simulink model "CACC_4_Robots"  (R2021a)
settings: Solver=FixedStepAuto  StartTime=0.0  StopTime=Tsim  RelTol=1e-3
values from neighbouring files (symbols this model uses):
  h = 1.0    (= 1)    [ros_cacc.m]    (also in ros_cacc2.m)
  k1 = 1    [ros_cacc.m]    (also in ros_cacc2.m)
  k2 = 1    [ros_cacc.m]    (also in ros_cacc2.m)
  r = 1    [ros_cacc.m]    (also in ros_cacc2.m)
  v_0 = 0.5    [ros_cacc.m]    (also in ros_cacc2.m)
  v_threshold = v_thr    (= 0.1)    [ros_cacc.m]    (also in ros_cacc2.m)
undefined symbols (not defined in the file or in its folder): angular, linear
libraries: ros2lib x17, robotcorelib x4
(part 2 of 3)

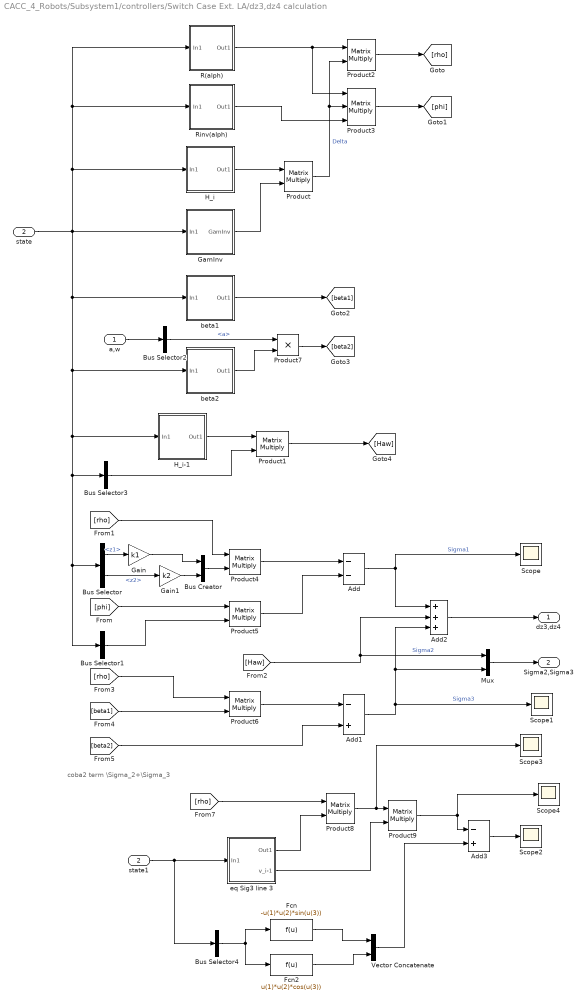
== system CACC_4_Robots/Subsystem1/controllers/Switch Case Ext. LA/dz3,dz4 calculation ==
  note: coba2 term \Sigma_2+\Sigma_3
  a,w : Inport
  state : Inport  Port=2
  Add : Sum  Inputs=--
  Add1 : Sum  Inputs=-+
  Add2 : Sum  Inputs=+++
  Add3 : Sum  Inputs=-+
  Bus Creator : BusCreator  Inputs=2
  Bus Selector : BusSelector  OutputSignals=z1,z2
  Bus Selector1 : BusSelector  OutputSignals=z3,z4  OutputAsBus=on
  Bus Selector2 : BusSelector  OutputSignals=a
  Bus Selector3 : BusSelector  OutputSignals=vdot_ref,thetadot_ref  OutputAsBus=on
  Bus Selector4 : BusSelector  OutputSignals=v_ref,thetadot_ref,theta_ref  OutputAsBus=on
  Fcn : Fcn  Expr=-u(1)*u(2)*sin(u(3))
  Fcn2 : Fcn  Expr=u(1)*u(2)*cos(u(3))
  Gain : Gain  Gain=k1
  Gain1 : Gain  Gain=k2
  "GamInv " : Subsystem
  H_i : Subsystem
  H_i-1 : Subsystem
  Mux : Mux  Inputs=2
  Product{,1..2,4..6,8..9} (8 alike) : Product  Multiplication=Matrix(*)
  Product3 : Product  Inputs=3  Multiplication=Matrix(*)
  Product7 : Product
  R(alph) : Subsystem
  Rinv(alph) : Subsystem
  Scope{,1..4} (5 alike) : Scope
  Vector Concatenate : Concatenate
  beta1 : Subsystem
  beta2 : Subsystem
  eq Sig3 line 3 : Subsystem
  state1 : InportShadow  Port=2
  dz3,dz4 : Outport  VectorParamsAs1DForOutWhenUnconnected=off
  Sigma2,Sigma3 : Outport  Port=2  VectorParamsAs1DForOutWhenUnconnected=off
  wires:
  state/1 -> beta1/1(In1), beta2/1(In1), H_i-1/1(In1), Bus Selector3/1, Bus Selector1/1, Bus Selector/1, Rinv(alph)/1(In1), R(alph)/1(In1), H_i/1(In1), "GamInv "/1(In1)
  H_i-1/1(Out1) -> Product1/1
  H_i/1(Out1) -> Product/1
  "GamInv "/1(GamInv) -> Product/2
  R(alph)/1(Out1) -> Product3/1, Product2/1
  Product/1 -> Product3/2, Product2/2  "Delta"
  Rinv(alph)/1(Out1) -> Product3/3
  Product2/1 -> [rho]
  Product3/1 -> [phi]
  beta1/1(Out1) -> [beta1]
  Product1/1 -> [Haw]
  Bus Selector/1 -> Gain/1  "<z1>"
  Bus Selector/2 -> Gain1/1  "<z2>"
  Gain/1 -> Bus Creator/1
  Gain1/1 -> Bus Creator/2
  Bus Creator/1 -> Product4/2
  [rho] -> Product4/1
  [phi] -> Product5/1
  Bus Selector1/1 -> Product5/2
  Product4/1 -> Add/1
  Product5/1 -> Add/2
  [rho] -> Product6/1
  [beta1] -> Product6/2
  Product6/1 -> Add1/1
  Add/1 -> Add2/1, Scope/1  "Sigma1"
  Add1/1 -> Mux/2, Add2/3, Scope1/1  "Sigma3"
  Add2/1 -> dz3,dz4/1
  a,w/1 -> Bus Selector2/1
  Bus Selector2/1 -> Product7/1  "<a>"
  [Haw] -> Mux/1, Add2/2  "Sigma2"
  Product7/1 -> [beta2]
  beta2/1(Out1) -> Product7/2
  [beta2] -> Add1/2
  Bus Selector3/1 -> Product1/2
  [rho] -> Product8/1
  eq Sig3 line 3/1(Out1) -> Product8/2
  Product8/1 -> Scope3/1, Product9/1
  Vector Concatenate/1 -> Add3/2
  Add3/1 -> Scope2/1
  state1/1 -> Bus Selector4/1, eq Sig3 line 3/1(In1)
  Bus Selector4/1 -> Fcn2/1, Fcn/1
  Fcn/1 -> Vector Concatenate/1
  Fcn2/1 -> Vector Concatenate/2
  eq Sig3 line 3/2(v_i-1) -> Product9/2
  Product9/1 -> Scope4/1, Add3/1
  Mux/1 -> Sigma2,Sigma3/1

== system CACC_4_Robots/Subsystem1/controllers/Switch Case Ext. LA/in parentheses ==
  In1 : Inport
  Add : Sum  Inputs=++++
  Bus Selector : BusSelector  OutputSignals=z1,z2
  Bus Selector1 : BusSelector  OutputSignals=alpha,z3,z4  OutputAsBus=on
  Bus Selector2 : BusSelector  OutputSignals=alpha,v_ref,theta_ref  OutputAsBus=on
  Bus Selector3 : BusSelector  OutputSignals=theta_ref,thetadot_ref,s  OutputAsBus=on
  Fcn : Fcn  Expr=cos(u(1))*u(2)+sin(u(1))*u(3)
  Fcn1 : Fcn  Expr=sin(u(1))*u(2)+cos(u(1))*u(3)
  Fcn2 : Fcn  Expr=(1-cos(u(1)))*u(2)*cos(u(3))-sin(u(1))*u(2)*sin(u(3))
  Fcn3 : Fcn  Expr=sin(u(1))*u(2)*cos(u(3))+(1-cos(u(1)))*u(2)*sin(u(3))
  Fcn4 : Fcn  Expr=cos(u(1))*u(3)*u(2)
  Fcn5 : Fcn  Expr=sin(u(1))*u(3)*u(2)
  Gain : Gain  Gain=k1
  Gain1 : Gain  Gain=k2
  Mux{1..4} (4 alike) : Mux  Inputs=2
  () : Outport  VectorParamsAs1DForOutWhenUnconnected=off
  wires:
  In1/1 -> Bus Selector3/1, Bus Selector2/1, Bus Selector1/1, Bus Selector/1
  Bus Selector/1 -> Gain/1  "<z1>"
  Bus Selector/2 -> Gain1/1  "<z2>"
  Gain/1 -> Mux1/1
  Gain1/1 -> Mux1/2
  Bus Selector1/1 -> Fcn1/1, Fcn/1
  Fcn/1 -> Mux2/1
  Fcn1/1 -> Mux2/2
  Bus Selector2/1 -> Fcn3/1, Fcn2/1
  Fcn2/1 -> Mux3/1
  Fcn3/1 -> Mux3/2
  Bus Selector3/1 -> Fcn5/1, Fcn4/1
  Fcn4/1 -> Mux4/1
  Fcn5/1 -> Mux4/2
  Mux1/1 -> Add/1
  Mux2/1 -> Add/2
  Mux3/1 -> Add/3
  Mux4/1 -> Add/4
  Add/1 -> ()/1

== system CACC_4_Robots/Subsystem1/controllers/Switch Case Ext. LA/invGam ==
  In1 : Inport
  11 : Fcn  Expr=(r+h*u(1))*cos(u(2))
  12 : Fcn  Expr=(r+h*u(1))*sin(u(2))
  21 : Fcn  Expr=-h*sin(u(2))-h*sin(u(13))*cos(u(8))
  22 : Fcn  Expr=h*cos(u(2))-h*sin(u(13))*sin(u(8))
  Divide{,1..3} (4 alike) : Product  Inputs=*/
  Mux : Mux
  det(Gam) : Fcn  Expr=((r+h*u(1))*(h-h*sin(u(13))*sin(u(8)-u(2))))
  invGam : Outport  VectorParamsAs1DForOutWhenUnconnected=off
  wires:
  In1/1 -> 11/1, 12/1, 22/1, det(Gam)/1, 21/1
  Mux/1 -> invGam/1
  11/1 -> Divide/1
  12/1 -> Divide1/1
  21/1 -> Divide2/1
  22/1 -> Divide3/1
  det(Gam)/1 -> Divide2/2, Divide1/2, Divide/2, Divide3/2
  Divide/1 -> Mux/1
  Divide1/1 -> Mux/2
  Divide2/1 -> Mux/3
  Divide3/1 -> Mux/4

== system CACC_4_Robots/Subsystem1/controllers/Switch Case Ext. LA/s ==
  state_prec : Inport
  state : Inport  Port=2
  Approximation of s around zero : Subsystem  TreatAsAtomicUnit=on
  Bus Selector : BusSelector  OutputSignals=curv
  Bus Selector1 : BusSelector  OutputSignals=v
  If : If  IfExpression=u1 < 0.01 & u1 > -0.01
  Merge : Merge
  Mux : Mux  Inputs=2
  function s : Subsystem  TreatAsAtomicUnit=on
  s : Outport  VectorParamsAs1DForOutWhenUnconnected=off
  wires:
  state_prec/1 -> Bus Selector/1
  Bus Selector/1 -> Mux/1, If/1  "<curv>"
  If/1 -> Approximation of s around zero/Action
  If/2 -> function s/Action
  Approximation of s around zero/1(Out1) -> Merge/1
  function s/1(Out1) -> Merge/2
  state/1 -> Bus Selector1/1
  Bus Selector1/1 -> Mux/2  "<v>"
  Mux/1 -> function s/1(In1), Approximation of s around zero/1(In1)
  Merge/1 -> s/1

== system CACC_4_Robots/Subsystem2/controllers/Switch Case Ext. LA/alpha ==
  state_prec : Inport
  state : Inport  Port=2
  Bus Selector : BusSelector  OutputSignals=curv
  Bus Selector1 : BusSelector  OutputSignals=v
  Fcn : Fcn  Expr=atan(u(1)*(r+h*u(2)))
  Mux : Mux  Inputs=2
  alpha : Outport  VectorParamsAs1DForOutWhenUnconnected=off
  wires:
  state_prec/1 -> Bus Selector/1
  state/1 -> Bus Selector1/1
  Mux/1 -> Fcn/1
  Bus Selector/1 -> Mux/1  "<curv>"
  Bus Selector1/1 -> Mux/2  "<v>"
  Fcn/1 -> alpha/1

== system CACC_4_Robots/Subsystem2/controllers/Switch Case Ext. LA/disturbance term simplified ==
  In1 : Inport
  (a,w)ref : Inport  Port=2
  Add : Sum  Inputs=-+
  "GamInv " : Subsystem
  H : Subsystem
  H1 : Subsystem
  Product : Product  Inputs=4  Multiplication=Matrix(*)
  Product1 : Product  Multiplication=Matrix(*)
  R(alph) : Subsystem
  beta1 : Subsystem
  dist1,dist2 : Outport  VectorParamsAs1DForOutWhenUnconnected=off
  wires:
  Add/1 -> dist1,dist2/1
  Product/1 -> Add/1
  (a,w)ref/1 -> Product1/2
  H1/1(Out1) -> Product1/1
  beta1/1(Out1) -> Product/4
  "GamInv "/1(GamInv) -> Product/3
  H/1(Out1) -> Product/2
  R(alph)/1(Out1) -> Product/1
  In1/1 -> H/1(In1), R(alph)/1(In1), "GamInv "/1(In1), beta1/1(In1), H1/1(In1)
  Product1/1 -> Add/2

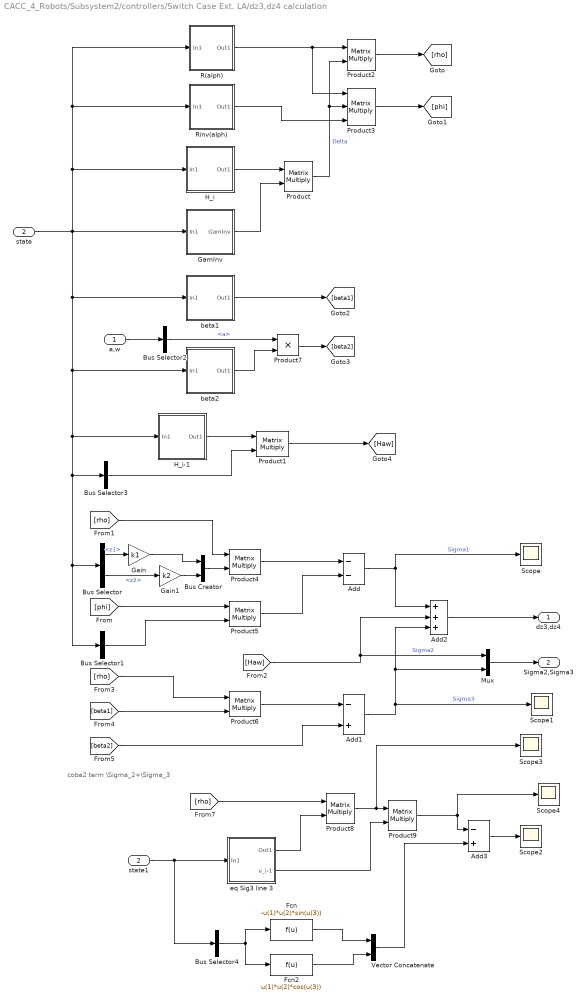
== system CACC_4_Robots/Subsystem2/controllers/Switch Case Ext. LA/dz3,dz4 calculation ==
  note: coba2 term \Sigma_2+\Sigma_3
  a,w : Inport
  state : Inport  Port=2
  Add : Sum  Inputs=--
  Add1 : Sum  Inputs=-+
  Add2 : Sum  Inputs=+++
  Add3 : Sum  Inputs=-+
  Bus Creator : BusCreator  Inputs=2
  Bus Selector : BusSelector  OutputSignals=z1,z2
  Bus Selector1 : BusSelector  OutputSignals=z3,z4  OutputAsBus=on
  Bus Selector2 : BusSelector  OutputSignals=a
  Bus Selector3 : BusSelector  OutputSignals=vdot_ref,thetadot_ref  OutputAsBus=on
  Bus Selector4 : BusSelector  OutputSignals=v_ref,thetadot_ref,theta_ref  OutputAsBus=on
  Fcn : Fcn  Expr=-u(1)*u(2)*sin(u(3))
  Fcn2 : Fcn  Expr=u(1)*u(2)*cos(u(3))
  Gain : Gain  Gain=k1
  Gain1 : Gain  Gain=k2
  "GamInv " : Subsystem
  H_i : Subsystem
  H_i-1 : Subsystem
  Mux : Mux  Inputs=2
  Product{,1..2,4..6,8..9} (8 alike) : Product  Multiplication=Matrix(*)
  Product3 : Product  Inputs=3  Multiplication=Matrix(*)
  Product7 : Product
  R(alph) : Subsystem
  Rinv(alph) : Subsystem
  Scope{,1..4} (5 alike) : Scope
  Vector Concatenate : Concatenate
  beta1 : Subsystem
  beta2 : Subsystem
  eq Sig3 line 3 : Subsystem
  state1 : InportShadow  Port=2
  dz3,dz4 : Outport  VectorParamsAs1DForOutWhenUnconnected=off
  Sigma2,Sigma3 : Outport  Port=2  VectorParamsAs1DForOutWhenUnconnected=off
  wires:
  state/1 -> beta1/1(In1), beta2/1(In1), H_i-1/1(In1), Bus Selector3/1, Bus Selector1/1, Bus Selector/1, Rinv(alph)/1(In1), R(alph)/1(In1), H_i/1(In1), "GamInv "/1(In1)
  H_i-1/1(Out1) -> Product1/1
  H_i/1(Out1) -> Product/1
  "GamInv "/1(GamInv) -> Product/2
  R(alph)/1(Out1) -> Product3/1, Product2/1
  Product/1 -> Product3/2, Product2/2  "Delta"
  Rinv(alph)/1(Out1) -> Product3/3
  Product2/1 -> [rho]
  Product3/1 -> [phi]
  beta1/1(Out1) -> [beta1]
  Product1/1 -> [Haw]
  Bus Selector/1 -> Gain/1  "<z1>"
  Bus Selector/2 -> Gain1/1  "<z2>"
  Gain/1 -> Bus Creator/1
  Gain1/1 -> Bus Creator/2
  Bus Creator/1 -> Product4/2
  [rho] -> Product4/1
  [phi] -> Product5/1
  Bus Selector1/1 -> Product5/2
  Product4/1 -> Add/1
  Product5/1 -> Add/2
  [rho] -> Product6/1
  [beta1] -> Product6/2
  Product6/1 -> Add1/1
  Add/1 -> Add2/1, Scope/1  "Sigma1"
  Add1/1 -> Mux/2, Add2/3, Scope1/1  "Sigma3"
  Add2/1 -> dz3,dz4/1
  a,w/1 -> Bus Selector2/1
  Bus Selector2/1 -> Product7/1  "<a>"
  [Haw] -> Mux/1, Add2/2  "Sigma2"
  Product7/1 -> [beta2]
  beta2/1(Out1) -> Product7/2
  [beta2] -> Add1/2
  Bus Selector3/1 -> Product1/2
  [rho] -> Product8/1
  eq Sig3 line 3/1(Out1) -> Product8/2
  Product8/1 -> Scope3/1, Product9/1
  Vector Concatenate/1 -> Add3/2
  Add3/1 -> Scope2/1
  state1/1 -> Bus Selector4/1, eq Sig3 line 3/1(In1)
  Bus Selector4/1 -> Fcn2/1, Fcn/1
  Fcn/1 -> Vector Concatenate/1
  Fcn2/1 -> Vector Concatenate/2
  eq Sig3 line 3/2(v_i-1) -> Product9/2
  Product9/1 -> Scope4/1, Add3/1
  Mux/1 -> Sigma2,Sigma3/1

== system CACC_4_Robots/Subsystem2/controllers/Switch Case Ext. LA/in parentheses ==
  In1 : Inport
  Add : Sum  Inputs=++++
  Bus Selector : BusSelector  OutputSignals=z1,z2
  Bus Selector1 : BusSelector  OutputSignals=alpha,z3,z4  OutputAsBus=on
  Bus Selector2 : BusSelector  OutputSignals=alpha,v_ref,theta_ref  OutputAsBus=on
  Bus Selector3 : BusSelector  OutputSignals=theta_ref,thetadot_ref,s  OutputAsBus=on
  Fcn : Fcn  Expr=cos(u(1))*u(2)+sin(u(1))*u(3)
  Fcn1 : Fcn  Expr=sin(u(1))*u(2)+cos(u(1))*u(3)
  Fcn2 : Fcn  Expr=(1-cos(u(1)))*u(2)*cos(u(3))-sin(u(1))*u(2)*sin(u(3))
  Fcn3 : Fcn  Expr=sin(u(1))*u(2)*cos(u(3))+(1-cos(u(1)))*u(2)*sin(u(3))
  Fcn4 : Fcn  Expr=cos(u(1))*u(3)*u(2)
  Fcn5 : Fcn  Expr=sin(u(1))*u(3)*u(2)
  Gain : Gain  Gain=k1
  Gain1 : Gain  Gain=k2
  Mux{1..4} (4 alike) : Mux  Inputs=2
  () : Outport  VectorParamsAs1DForOutWhenUnconnected=off
  wires:
  In1/1 -> Bus Selector3/1, Bus Selector2/1, Bus Selector1/1, Bus Selector/1
  Bus Selector/1 -> Gain/1  "<z1>"
  Bus Selector/2 -> Gain1/1  "<z2>"
  Gain/1 -> Mux1/1
  Gain1/1 -> Mux1/2
  Bus Selector1/1 -> Fcn1/1, Fcn/1
  Fcn/1 -> Mux2/1
  Fcn1/1 -> Mux2/2
  Bus Selector2/1 -> Fcn3/1, Fcn2/1
  Fcn2/1 -> Mux3/1
  Fcn3/1 -> Mux3/2
  Bus Selector3/1 -> Fcn5/1, Fcn4/1
  Fcn4/1 -> Mux4/1
  Fcn5/1 -> Mux4/2
  Mux1/1 -> Add/1
  Mux2/1 -> Add/2
  Mux3/1 -> Add/3
  Mux4/1 -> Add/4
  Add/1 -> ()/1

== system CACC_4_Robots/Subsystem2/controllers/Switch Case Ext. LA/invGam ==
  In1 : Inport
  11 : Fcn  Expr=(r+h*u(1))*cos(u(2))
  12 : Fcn  Expr=(r+h*u(1))*sin(u(2))
  21 : Fcn  Expr=-h*sin(u(2))-h*sin(u(13))*cos(u(8))
  22 : Fcn  Expr=h*cos(u(2))-h*sin(u(13))*sin(u(8))
  Divide{,1..3} (4 alike) : Product  Inputs=*/
  Mux : Mux
  det(Gam) : Fcn  Expr=((r+h*u(1))*(h-h*sin(u(13))*sin(u(8)-u(2))))
  invGam : Outport  VectorParamsAs1DForOutWhenUnconnected=off
  wires:
  In1/1 -> 11/1, 12/1, 22/1, det(Gam)/1, 21/1
  Mux/1 -> invGam/1
  11/1 -> Divide/1
  12/1 -> Divide1/1
  21/1 -> Divide2/1
  22/1 -> Divide3/1
  det(Gam)/1 -> Divide2/2, Divide1/2, Divide/2, Divide3/2
  Divide/1 -> Mux/1
  Divide1/1 -> Mux/2
  Divide2/1 -> Mux/3
  Divide3/1 -> Mux/4

== system CACC_4_Robots/Subsystem2/controllers/Switch Case Ext. LA/s ==
  state_prec : Inport
  state : Inport  Port=2
  Approximation of s around zero : Subsystem  TreatAsAtomicUnit=on
  Bus Selector : BusSelector  OutputSignals=curv
  Bus Selector1 : BusSelector  OutputSignals=v
  If : If  IfExpression=u1 < 0.01 & u1 > -0.01
  Merge : Merge
  Mux : Mux  Inputs=2
  function s : Subsystem  TreatAsAtomicUnit=on
  s : Outport  VectorParamsAs1DForOutWhenUnconnected=off
  wires:
  state_prec/1 -> Bus Selector/1
  Bus Selector/1 -> Mux/1, If/1  "<curv>"
  If/1 -> Approximation of s around zero/Action
  If/2 -> function s/Action
  Approximation of s around zero/1(Out1) -> Merge/1
  function s/1(Out1) -> Merge/2
  state/1 -> Bus Selector1/1
  Bus Selector1/1 -> Mux/2  "<v>"
  Mux/1 -> function s/1(In1), Approximation of s around zero/1(In1)
  Merge/1 -> s/1

== system CACC_4_Robots/Subsystem/controllers/Switch Case Ext. LA/disturbance term simplified/GamInv  ==
  In1 : Inport
  11 : Fcn  Expr=(r+h*u(1))*cos(u(2))
  12 : Fcn  Expr=(r+h*u(1))*sin(u(2))
  21 : Fcn  Expr=-h*sin(u(2))-h*sin(u(13))*cos(u(8))
  22 : Fcn  Expr=h*cos(u(2))-h*sin(u(13))*sin(u(8))
  Divide{,1..3} (4 alike) : Product  Inputs=*/
  Vector Concatenate : Concatenate
  Vector Concatenate1 : Concatenate
  Vector Concatenate2 : Concatenate  Mode=Multidimensional array  ConcatenateDimension=2
  det(Gam) : Fcn  Expr=((r+h*u(1))*(h-h*sin(u(13))*sin(u(8)-u(2))))
  GamInv : Outport  VectorParamsAs1DForOutWhenUnconnected=off
  wires:
  Vector Concatenate2/1 -> GamInv/1
  Vector Concatenate1/1 -> Vector Concatenate2/2
  Vector Concatenate/1 -> Vector Concatenate2/1
  Divide3/1 -> Vector Concatenate1/2
  Divide1/1 -> Vector Concatenate1/1
  Divide2/1 -> Vector Concatenate/2
  Divide/1 -> Vector Concatenate/1
  In1/1 -> 11/1, 12/1, 21/1, 22/1, det(Gam)/1
  det(Gam)/1 -> Divide3/2, Divide/2, Divide1/2, Divide2/2
  22/1 -> Divide3/1
  21/1 -> Divide2/1
  12/1 -> Divide1/1
  11/1 -> Divide/1

== system CACC_4_Robots/Subsystem/controllers/Switch Case Ext. LA/disturbance term simplified/H ==
  In1 : Inport
  Bus Selector1 : BusSelector  OutputSignals=v,theta  OutputAsBus=on
  H11 : Fcn  Expr=cos(u(2))
  H12 : Fcn  Expr=-u(1)*sin(u(2))
  H21 : Fcn  Expr=sin(u(2))
  H22 : Fcn  Expr=u(1)*cos(u(2))
  Vector Concatenate3 : Concatenate
  Vector Concatenate4 : Concatenate
  Vector Concatenate5 : Concatenate  Mode=Multidimensional array  ConcatenateDimension=2
  Out1 : Outport  VectorParamsAs1DForOutWhenUnconnected=off
  wires:
  Vector Concatenate5/1 -> Out1/1
  H22/1 -> Vector Concatenate4/2
  H12/1 -> Vector Concatenate4/1
  H21/1 -> Vector Concatenate3/2
  H11/1 -> Vector Concatenate3/1
  Vector Concatenate4/1 -> Vector Concatenate5/2
  Vector Concatenate3/1 -> Vector Concatenate5/1
  In1/1 -> Bus Selector1/1
  Bus Selector1/1 -> H12/1, H21/1, H22/1, H11/1

== system CACC_4_Robots/Subsystem/controllers/Switch Case Ext. LA/disturbance term simplified/H1 ==
  In1 : Inport
  Bus Selector1 : BusSelector  OutputSignals=v,theta  OutputAsBus=on
  H11 : Fcn  Expr=cos(u(2))
  H12 : Fcn  Expr=-u(1)*sin(u(2))
  H21 : Fcn  Expr=sin(u(2))
  H22 : Fcn  Expr=u(1)*cos(u(2))
  Vector Concatenate3 : Concatenate
  Vector Concatenate4 : Concatenate
  Vector Concatenate5 : Concatenate  Mode=Multidimensional array  ConcatenateDimension=2
  Out1 : Outport  VectorParamsAs1DForOutWhenUnconnected=off
  wires:
  Bus Selector1/1 -> H11/1, H22/1, H21/1, H12/1
  In1/1 -> Bus Selector1/1
  Vector Concatenate3/1 -> Vector Concatenate5/1
  Vector Concatenate4/1 -> Vector Concatenate5/2
  H11/1 -> Vector Concatenate3/1
  H21/1 -> Vector Concatenate3/2
  H12/1 -> Vector Concatenate4/1
  H22/1 -> Vector Concatenate4/2
  Vector Concatenate5/1 -> Out1/1

== system CACC_4_Robots/Subsystem/controllers/Switch Case Ext. LA/disturbance term simplified/R(alph) ==
  In1 : Inport
  Bus Selector : BusSelector  OutputSignals=alpha
  R11 : Fcn  Expr=cos(u(1))
  R12 : Fcn  Expr=-sin(u(1))
  R21 : Fcn  Expr=sin(u(1))
  R22 : Fcn  Expr=cos(u(1))
  Vector Concatenate6 : Concatenate
  Vector Concatenate7 : Concatenate
  Vector Concatenate8 : Concatenate  Mode=Multidimensional array  ConcatenateDimension=2
  Out1 : Outport  VectorParamsAs1DForOutWhenUnconnected=off
  wires:
  Vector Concatenate8/1 -> Out1/1
  R22/1 -> Vector Concatenate7/2
  R12/1 -> Vector Concatenate7/1
  R21/1 -> Vector Concatenate6/2
  R11/1 -> Vector Concatenate6/1
  Vector Concatenate7/1 -> Vector Concatenate8/2
  Vector Concatenate6/1 -> Vector Concatenate8/1
  Bus Selector/1 -> R22/1, R21/1, R12/1, R11/1  "<alpha>"
  In1/1 -> Bus Selector/1

== system CACC_4_Robots/Subsystem/controllers/Switch Case Ext. LA/disturbance term simplified/beta1 ==
  In1 : Inport
  1 : Fcn  Expr=u(1)*cos(u(2))
  11 : Fcn  Expr=u(2)*(r+h*u(1))*sin(u(3))
  12 : Fcn  Expr=-sin(u(3))
  2 : Fcn  Expr=u(1)*sin(u(2))
  Bus Selector : BusSelector  OutputSignals=v,curv,alpha  OutputAsBus=on
  Bus Selector1 : BusSelector  OutputSignals=v_ref,theta_ref  OutputAsBus=on
  Product : Product  Multiplication=Matrix(*)
  Vector Concatenate : Concatenate
  Vector Concatenate1 : Concatenate
  Vector Concatenate2 : Concatenate  Mode=Multidimensional array  ConcatenateDimension=2
  Vector Concatenate3 : Concatenate
  Out1 : Outport  VectorParamsAs1DForOutWhenUnconnected=off
  wires:
  In1/1 -> Bus Selector1/1, Bus Selector/1
  Bus Selector/1 -> 11/1, 12/1
  11/1 -> Vector Concatenate1/2, Vector Concatenate/1
  12/1 -> Vector Concatenate1/1, Vector Concatenate/2
  Vector Concatenate/1 -> Vector Concatenate2/1
  Vector Concatenate1/1 -> Vector Concatenate2/2
  1/1 -> Vector Concatenate3/1
  2/1 -> Vector Concatenate3/2
  Bus Selector1/1 -> 2/1, 1/1
  Vector Concatenate2/1 -> Product/1
  Vector Concatenate3/1 -> Product/2
  Product/1 -> Out1/1

== system CACC_4_Robots/Subsystem/controllers/Switch Case Ext. LA/dz3,dz4 calculation/GamInv  ==
  In1 : Inport
  11 : Fcn  Expr=(r+h*u(1))*cos(u(2))
  12 : Fcn  Expr=(r+h*u(1))*sin(u(2))
  21 : Fcn  Expr=-h*sin(u(2))-h*sin(u(13))*cos(u(8))
  22 : Fcn  Expr=h*cos(u(2))-h*sin(u(13))*sin(u(8))
  Divide{,1..3} (4 alike) : Product  Inputs=*/
  Vector Concatenate : Concatenate
  Vector Concatenate1 : Concatenate
  Vector Concatenate2 : Concatenate  Mode=Multidimensional array  ConcatenateDimension=2
  det(Gam) : Fcn  Expr=((r+h*u(1))*(h-h*sin(u(13))*sin(u(8)-u(2))))
  GamInv : Outport  VectorParamsAs1DForOutWhenUnconnected=off
  wires:
  11/1 -> Divide/1
  12/1 -> Divide1/1
  21/1 -> Divide2/1
  22/1 -> Divide3/1
  det(Gam)/1 -> Divide2/2, Divide1/2, Divide/2, Divide3/2
  In1/1 -> det(Gam)/1, 22/1, 21/1, 12/1, 11/1
  Divide/1 -> Vector Concatenate/1
  Divide2/1 -> Vector Concatenate/2
  Divide1/1 -> Vector Concatenate1/1
  Divide3/1 -> Vector Concatenate1/2
  Vector Concatenate/1 -> Vector Concatenate2/1
  Vector Concatenate1/1 -> Vector Concatenate2/2
  Vector Concatenate2/1 -> GamInv/1

== system CACC_4_Robots/Subsystem/controllers/Switch Case Ext. LA/dz3,dz4 calculation/H_i ==
  In1 : Inport
  Bus Selector1 : BusSelector  OutputSignals=v,theta  OutputAsBus=on
  H11 : Fcn  Expr=cos(u(2))
  H12 : Fcn  Expr=-u(1)*sin(u(2))
  H21 : Fcn  Expr=sin(u(2))
  H22 : Fcn  Expr=u(1)*cos(u(2))
  Vector Concatenate3 : Concatenate
  Vector Concatenate4 : Concatenate
  Vector Concatenate5 : Concatenate  Mode=Multidimensional array  ConcatenateDimension=2
  Out1 : Outport  VectorParamsAs1DForOutWhenUnconnected=off
  wires:
  Bus Selector1/1 -> H11/1, H22/1, H21/1, H12/1
  In1/1 -> Bus Selector1/1
  Vector Concatenate3/1 -> Vector Concatenate5/1
  Vector Concatenate4/1 -> Vector Concatenate5/2
  H11/1 -> Vector Concatenate3/1
  H21/1 -> Vector Concatenate3/2
  H12/1 -> Vector Concatenate4/1
  H22/1 -> Vector Concatenate4/2
  Vector Concatenate5/1 -> Out1/1

== system CACC_4_Robots/Subsystem/controllers/Switch Case Ext. LA/dz3,dz4 calculation/H_i-1 ==
  In1 : Inport
  Bus Selector1 : BusSelector  OutputSignals=v_ref,theta_ref  OutputAsBus=on
  H11 : Fcn  Expr=cos(u(2))
  H12 : Fcn  Expr=-u(1)*sin(u(2))
  H21 : Fcn  Expr=sin(u(2))
  H22 : Fcn  Expr=u(1)*cos(u(2))
  Vector Concatenate3 : Concatenate
  Vector Concatenate4 : Concatenate
  Vector Concatenate5 : Concatenate  Mode=Multidimensional array  ConcatenateDimension=2
  Out1 : Outport  VectorParamsAs1DForOutWhenUnconnected=off
  wires:
  Vector Concatenate5/1 -> Out1/1
  H22/1 -> Vector Concatenate4/2
  H12/1 -> Vector Concatenate4/1
  H21/1 -> Vector Concatenate3/2
  H11/1 -> Vector Concatenate3/1
  Vector Concatenate4/1 -> Vector Concatenate5/2
  Vector Concatenate3/1 -> Vector Concatenate5/1
  In1/1 -> Bus Selector1/1
  Bus Selector1/1 -> H12/1, H21/1, H22/1, H11/1

== system CACC_4_Robots/Subsystem/controllers/Switch Case Ext. LA/dz3,dz4 calculation/R(alph) ==
  In1 : Inport
  Bus Selector : BusSelector  OutputSignals=alpha
  R11 : Fcn  Expr=cos(u(1))
  R12 : Fcn  Expr=-sin(u(1))
  R21 : Fcn  Expr=sin(u(1))
  R22 : Fcn  Expr=cos(u(1))
  Vector Concatenate6 : Concatenate
  Vector Concatenate7 : Concatenate
  Vector Concatenate8 : Concatenate  Mode=Multidimensional array  ConcatenateDimension=2
  Out1 : Outport  VectorParamsAs1DForOutWhenUnconnected=off
  wires:
  In1/1 -> Bus Selector/1
  Bus Selector/1 -> R11/1, R12/1, R21/1, R22/1  "<alpha>"
  Vector Concatenate6/1 -> Vector Concatenate8/1
  Vector Concatenate7/1 -> Vector Concatenate8/2
  R11/1 -> Vector Concatenate6/1
  R21/1 -> Vector Concatenate6/2
  R12/1 -> Vector Concatenate7/1
  R22/1 -> Vector Concatenate7/2
  Vector Concatenate8/1 -> Out1/1

== system CACC_4_Robots/Subsystem/controllers/Switch Case Ext. LA/dz3,dz4 calculation/Rinv(alph) ==
  In1 : Inport
  Bus Selector : BusSelector  OutputSignals=alpha
  R11 : Fcn  Expr=cos(u(1))
  R12 : Fcn  Expr=sin(u(1))
  R21 : Fcn  Expr=-sin(u(1))
  R22 : Fcn  Expr=cos(u(1))
  Vector Concatenate6 : Concatenate
  Vector Concatenate7 : Concatenate
  Vector Concatenate8 : Concatenate  Mode=Multidimensional array  ConcatenateDimension=2
  Out1 : Outport  VectorParamsAs1DForOutWhenUnconnected=off
  wires:
  Vector Concatenate8/1 -> Out1/1
  R22/1 -> Vector Concatenate7/2
  R12/1 -> Vector Concatenate7/1
  R21/1 -> Vector Concatenate6/2
  R11/1 -> Vector Concatenate6/1
  Vector Concatenate7/1 -> Vector Concatenate8/2
  Vector Concatenate6/1 -> Vector Concatenate8/1
  Bus Selector/1 -> R22/1, R21/1, R12/1, R11/1  "<alpha>"
  In1/1 -> Bus Selector/1

== system CACC_4_Robots/Subsystem/controllers/Switch Case Ext. LA/dz3,dz4 calculation/beta1 ==
  In1 : Inport
  Add : Sum
  Bus Selector2 : BusSelector  OutputSignals=alpha,v_ref,theta_ref  OutputAsBus=on
  Bus Selector3 : BusSelector  OutputSignals=theta_ref,thetadot_ref,s  OutputAsBus=on
  Fcn2 : Fcn  Expr=(1-cos(u(1)))*u(2)*cos(u(3))-sin(u(1))*u(2)*sin(u(3))
  Fcn3 : Fcn  Expr=sin(u(1))*u(2)*cos(u(3))+(1-cos(u(1)))*u(2)*sin(u(3))
  Fcn4 : Fcn  Expr=cos(u(1))*u(3)*u(2)
  Fcn5 : Fcn  Expr=sin(u(1))*u(3)*u(2)
  Mux3 : Mux  Inputs=2
  Mux4 : Mux  Inputs=2
  Out1 : Outport  VectorParamsAs1DForOutWhenUnconnected=off
  wires:
  Bus Selector2/1 -> Fcn3/1, Fcn2/1
  Fcn2/1 -> Mux3/1
  Fcn3/1 -> Mux3/2
  Bus Selector3/1 -> Fcn5/1, Fcn4/1
  Fcn4/1 -> Mux4/1
  Fcn5/1 -> Mux4/2
  Mux3/1 -> Add/1
  Mux4/1 -> Add/2
  In1/1 -> Bus Selector3/1, Bus Selector2/1
  Add/1 -> Out1/1

== system CACC_4_Robots/Subsystem/controllers/Switch Case Ext. LA/dz3,dz4 calculation/beta2 ==
  In1 : Inport
  Bus Selector : BusSelector  OutputSignals=v,theta,alpha,curv  OutputAsBus=on
  Mux : Mux  Inputs=2
  beta2_1 : Fcn  Expr=-u(1)*sin(u(2)+u(3))*(h*u(4)*cos(u(3))^2)
  beta2_2 : Fcn  Expr=u(1)*cos(u(2)+u(3))*(h*u(4)*cos(u(3))^2)
  Out1 : Outport  VectorParamsAs1DForOutWhenUnconnected=off
  wires:
  In1/1 -> Bus Selector/1
  Bus Selector/1 -> beta2_2/1, beta2_1/1
  beta2_1/1 -> Mux/1
  beta2_2/1 -> Mux/2
  Mux/1 -> Out1/1

== system CACC_4_Robots/Subsystem/controllers/Switch Case Ext. LA/dz3,dz4 calculation/eq Sig3 line 3 ==
  In1 : Inport
  1 : Fcn  Expr=u(1)*cos(u(2))
  2 : Fcn  Expr=u(1)*sin(u(2))
  Bus Selector1 : BusSelector  OutputSignals=v_ref,theta_ref  OutputAsBus=on
  Vector Concatenate3 : Concatenate
  mat : Subsystem
  Out1 : Outport  VectorParamsAs1DForOutWhenUnconnected=off
  v_i-1 : Outport  Port=2  VectorParamsAs1DForOutWhenUnconnected=off
  wires:
  In1/1 -> mat/1(In1), Bus Selector1/1
  Bus Selector1/1 -> 2/1, 1/1
  1/1 -> Vector Concatenate3/1
  2/1 -> Vector Concatenate3/2
  mat/1(Out1) -> Out1/1
  Vector Concatenate3/1 -> v_i-1/1

== system CACC_4_Robots/Subsystem/controllers/Switch Case Ext. LA/s/Approximation of s around zero ==
  In1 : Inport
  Action Port : ActionPort  ActionPortLabel=if(u1 < 0.01 & u1 > -0.01)
  Taylor approximation 3rd order : Fcn  Expr=0.5*(r+h*u(2))^2*u(1)-0.125*(r+h*u(2))^4*u(1)^3
  Out1 : Outport  VectorParamsAs1DForOutWhenUnconnected=off
  wires:
  In1/1 -> Taylor approximation 3rd order/1
  Taylor approximation 3rd order/1 -> Out1/1

== system CACC_4_Robots/Subsystem/controllers/Switch Case Ext. LA/s/function s ==
  In1 : Inport
  Action Port : ActionPort  ActionPortLabel=else
  function s : Fcn  Expr=(-1+sqrt(1+u(1)^2*(r+h*u(2))^2))/u(1)
  Out1 : Outport  VectorParamsAs1DForOutWhenUnconnected=off
  wires:
  In1/1 -> function s/1
  function s/1 -> Out1/1

== system CACC_4_Robots/Subsystem1/controllers/Switch Case Ext. LA/disturbance term simplified/GamInv  ==
  In1 : Inport
  11 : Fcn  Expr=(r+h*u(1))*cos(u(2))
  12 : Fcn  Expr=(r+h*u(1))*sin(u(2))
  21 : Fcn  Expr=-h*sin(u(2))-h*sin(u(13))*cos(u(8))
  22 : Fcn  Expr=h*cos(u(2))-h*sin(u(13))*sin(u(8))
  Divide{,1..3} (4 alike) : Product  Inputs=*/
  Vector Concatenate : Concatenate
  Vector Concatenate1 : Concatenate
  Vector Concatenate2 : Concatenate  Mode=Multidimensional array  ConcatenateDimension=2
  det(Gam) : Fcn  Expr=((r+h*u(1))*(h-h*sin(u(13))*sin(u(8)-u(2))))
  GamInv : Outport  VectorParamsAs1DForOutWhenUnconnected=off
  wires:
  Vector Concatenate2/1 -> GamInv/1
  Vector Concatenate1/1 -> Vector Concatenate2/2
  Vector Concatenate/1 -> Vector Concatenate2/1
  Divide3/1 -> Vector Concatenate1/2
  Divide1/1 -> Vector Concatenate1/1
  Divide2/1 -> Vector Concatenate/2
  Divide/1 -> Vector Concatenate/1
  In1/1 -> 11/1, 12/1, 21/1, 22/1, det(Gam)/1
  det(Gam)/1 -> Divide3/2, Divide/2, Divide1/2, Divide2/2
  22/1 -> Divide3/1
  21/1 -> Divide2/1
  12/1 -> Divide1/1
  11/1 -> Divide/1

== system CACC_4_Robots/Subsystem1/controllers/Switch Case Ext. LA/disturbance term simplified/H ==
  In1 : Inport
  Bus Selector1 : BusSelector  OutputSignals=v,theta  OutputAsBus=on
  H11 : Fcn  Expr=cos(u(2))
  H12 : Fcn  Expr=-u(1)*sin(u(2))
  H21 : Fcn  Expr=sin(u(2))
  H22 : Fcn  Expr=u(1)*cos(u(2))
  Vector Concatenate3 : Concatenate
  Vector Concatenate4 : Concatenate
  Vector Concatenate5 : Concatenate  Mode=Multidimensional array  ConcatenateDimension=2
  Out1 : Outport  VectorParamsAs1DForOutWhenUnconnected=off
  wires:
  Vector Concatenate5/1 -> Out1/1
  H22/1 -> Vector Concatenate4/2
  H12/1 -> Vector Concatenate4/1
  H21/1 -> Vector Concatenate3/2
  H11/1 -> Vector Concatenate3/1
  Vector Concatenate4/1 -> Vector Concatenate5/2
  Vector Concatenate3/1 -> Vector Concatenate5/1
  In1/1 -> Bus Selector1/1
  Bus Selector1/1 -> H12/1, H21/1, H22/1, H11/1

== system CACC_4_Robots/Subsystem1/controllers/Switch Case Ext. LA/disturbance term simplified/H1 ==
  In1 : Inport
  Bus Selector1 : BusSelector  OutputSignals=v,theta  OutputAsBus=on
  H11 : Fcn  Expr=cos(u(2))
  H12 : Fcn  Expr=-u(1)*sin(u(2))
  H21 : Fcn  Expr=sin(u(2))
  H22 : Fcn  Expr=u(1)*cos(u(2))
  Vector Concatenate3 : Concatenate
  Vector Concatenate4 : Concatenate
  Vector Concatenate5 : Concatenate  Mode=Multidimensional array  ConcatenateDimension=2
  Out1 : Outport  VectorParamsAs1DForOutWhenUnconnected=off
  wires:
  Bus Selector1/1 -> H11/1, H22/1, H21/1, H12/1
  In1/1 -> Bus Selector1/1
  Vector Concatenate3/1 -> Vector Concatenate5/1
  Vector Concatenate4/1 -> Vector Concatenate5/2
  H11/1 -> Vector Concatenate3/1
  H21/1 -> Vector Concatenate3/2
  H12/1 -> Vector Concatenate4/1
  H22/1 -> Vector Concatenate4/2
  Vector Concatenate5/1 -> Out1/1

== system CACC_4_Robots/Subsystem1/controllers/Switch Case Ext. LA/disturbance term simplified/R(alph) ==
  In1 : Inport
  Bus Selector : BusSelector  OutputSignals=alpha
  R11 : Fcn  Expr=cos(u(1))
  R12 : Fcn  Expr=-sin(u(1))
  R21 : Fcn  Expr=sin(u(1))
  R22 : Fcn  Expr=cos(u(1))
  Vector Concatenate6 : Concatenate
  Vector Concatenate7 : Concatenate
  Vector Concatenate8 : Concatenate  Mode=Multidimensional array  ConcatenateDimension=2
  Out1 : Outport  VectorParamsAs1DForOutWhenUnconnected=off
  wires:
  Vector Concatenate8/1 -> Out1/1
  R22/1 -> Vector Concatenate7/2
  R12/1 -> Vector Concatenate7/1
  R21/1 -> Vector Concatenate6/2
  R11/1 -> Vector Concatenate6/1
  Vector Concatenate7/1 -> Vector Concatenate8/2
  Vector Concatenate6/1 -> Vector Concatenate8/1
  Bus Selector/1 -> R22/1, R21/1, R12/1, R11/1  "<alpha>"
  In1/1 -> Bus Selector/1

== system CACC_4_Robots/Subsystem1/controllers/Switch Case Ext. LA/disturbance term simplified/beta1 ==
  In1 : Inport
  1 : Fcn  Expr=u(1)*cos(u(2))
  11 : Fcn  Expr=u(2)*(r+h*u(1))*sin(u(3))
  12 : Fcn  Expr=-sin(u(3))
  2 : Fcn  Expr=u(1)*sin(u(2))
  Bus Selector : BusSelector  OutputSignals=v,curv,alpha  OutputAsBus=on
  Bus Selector1 : BusSelector  OutputSignals=v_ref,theta_ref  OutputAsBus=on
  Product : Product  Multiplication=Matrix(*)
  Vector Concatenate : Concatenate
  Vector Concatenate1 : Concatenate
  Vector Concatenate2 : Concatenate  Mode=Multidimensional array  ConcatenateDimension=2
  Vector Concatenate3 : Concatenate
  Out1 : Outport  VectorParamsAs1DForOutWhenUnconnected=off
  wires:
  In1/1 -> Bus Selector1/1, Bus Selector/1
  Bus Selector/1 -> 11/1, 12/1
  11/1 -> Vector Concatenate1/2, Vector Concatenate/1
  12/1 -> Vector Concatenate1/1, Vector Concatenate/2
  Vector Concatenate/1 -> Vector Concatenate2/1
  Vector Concatenate1/1 -> Vector Concatenate2/2
  1/1 -> Vector Concatenate3/1
  2/1 -> Vector Concatenate3/2
  Bus Selector1/1 -> 2/1, 1/1
  Vector Concatenate2/1 -> Product/1
  Vector Concatenate3/1 -> Product/2
  Product/1 -> Out1/1

== system CACC_4_Robots/Subsystem1/controllers/Switch Case Ext. LA/dz3,dz4 calculation/GamInv  ==
  In1 : Inport
  11 : Fcn  Expr=(r+h*u(1))*cos(u(2))
  12 : Fcn  Expr=(r+h*u(1))*sin(u(2))
  21 : Fcn  Expr=-h*sin(u(2))-h*sin(u(13))*cos(u(8))
  22 : Fcn  Expr=h*cos(u(2))-h*sin(u(13))*sin(u(8))
  Divide{,1..3} (4 alike) : Product  Inputs=*/
  Vector Concatenate : Concatenate
  Vector Concatenate1 : Concatenate
  Vector Concatenate2 : Concatenate  Mode=Multidimensional array  ConcatenateDimension=2
  det(Gam) : Fcn  Expr=((r+h*u(1))*(h-h*sin(u(13))*sin(u(8)-u(2))))
  GamInv : Outport  VectorParamsAs1DForOutWhenUnconnected=off
  wires:
  11/1 -> Divide/1
  12/1 -> Divide1/1
  21/1 -> Divide2/1
  22/1 -> Divide3/1
  det(Gam)/1 -> Divide2/2, Divide1/2, Divide/2, Divide3/2
  In1/1 -> det(Gam)/1, 22/1, 21/1, 12/1, 11/1
  Divide/1 -> Vector Concatenate/1
  Divide2/1 -> Vector Concatenate/2
  Divide1/1 -> Vector Concatenate1/1
  Divide3/1 -> Vector Concatenate1/2
  Vector Concatenate/1 -> Vector Concatenate2/1
  Vector Concatenate1/1 -> Vector Concatenate2/2
  Vector Concatenate2/1 -> GamInv/1

== system CACC_4_Robots/Subsystem1/controllers/Switch Case Ext. LA/dz3,dz4 calculation/H_i ==
  In1 : Inport
  Bus Selector1 : BusSelector  OutputSignals=v,theta  OutputAsBus=on
  H11 : Fcn  Expr=cos(u(2))
  H12 : Fcn  Expr=-u(1)*sin(u(2))
  H21 : Fcn  Expr=sin(u(2))
  H22 : Fcn  Expr=u(1)*cos(u(2))
  Vector Concatenate3 : Concatenate
  Vector Concatenate4 : Concatenate
  Vector Concatenate5 : Concatenate  Mode=Multidimensional array  ConcatenateDimension=2
  Out1 : Outport  VectorParamsAs1DForOutWhenUnconnected=off
  wires:
  Bus Selector1/1 -> H11/1, H22/1, H21/1, H12/1
  In1/1 -> Bus Selector1/1
  Vector Concatenate3/1 -> Vector Concatenate5/1
  Vector Concatenate4/1 -> Vector Concatenate5/2
  H11/1 -> Vector Concatenate3/1
  H21/1 -> Vector Concatenate3/2
  H12/1 -> Vector Concatenate4/1
  H22/1 -> Vector Concatenate4/2
  Vector Concatenate5/1 -> Out1/1

== system CACC_4_Robots/Subsystem1/controllers/Switch Case Ext. LA/dz3,dz4 calculation/H_i-1 ==
  In1 : Inport
  Bus Selector1 : BusSelector  OutputSignals=v_ref,theta_ref  OutputAsBus=on
  H11 : Fcn  Expr=cos(u(2))
  H12 : Fcn  Expr=-u(1)*sin(u(2))
  H21 : Fcn  Expr=sin(u(2))
  H22 : Fcn  Expr=u(1)*cos(u(2))
  Vector Concatenate3 : Concatenate
  Vector Concatenate4 : Concatenate
  Vector Concatenate5 : Concatenate  Mode=Multidimensional array  ConcatenateDimension=2
  Out1 : Outport  VectorParamsAs1DForOutWhenUnconnected=off
  wires:
  Vector Concatenate5/1 -> Out1/1
  H22/1 -> Vector Concatenate4/2
  H12/1 -> Vector Concatenate4/1
  H21/1 -> Vector Concatenate3/2
  H11/1 -> Vector Concatenate3/1
  Vector Concatenate4/1 -> Vector Concatenate5/2
  Vector Concatenate3/1 -> Vector Concatenate5/1
  In1/1 -> Bus Selector1/1
  Bus Selector1/1 -> H12/1, H21/1, H22/1, H11/1

== system CACC_4_Robots/Subsystem1/controllers/Switch Case Ext. LA/dz3,dz4 calculation/R(alph) ==
  In1 : Inport
  Bus Selector : BusSelector  OutputSignals=alpha
  R11 : Fcn  Expr=cos(u(1))
  R12 : Fcn  Expr=-sin(u(1))
  R21 : Fcn  Expr=sin(u(1))
  R22 : Fcn  Expr=cos(u(1))
  Vector Concatenate6 : Concatenate
  Vector Concatenate7 : Concatenate
  Vector Concatenate8 : Concatenate  Mode=Multidimensional array  ConcatenateDimension=2
  Out1 : Outport  VectorParamsAs1DForOutWhenUnconnected=off
  wires:
  In1/1 -> Bus Selector/1
  Bus Selector/1 -> R11/1, R12/1, R21/1, R22/1  "<alpha>"
  Vector Concatenate6/1 -> Vector Concatenate8/1
  Vector Concatenate7/1 -> Vector Concatenate8/2
  R11/1 -> Vector Concatenate6/1
  R21/1 -> Vector Concatenate6/2
  R12/1 -> Vector Concatenate7/1
  R22/1 -> Vector Concatenate7/2
  Vector Concatenate8/1 -> Out1/1

== system CACC_4_Robots/Subsystem1/controllers/Switch Case Ext. LA/dz3,dz4 calculation/Rinv(alph) ==
  In1 : Inport
  Bus Selector : BusSelector  OutputSignals=alpha
  R11 : Fcn  Expr=cos(u(1))
  R12 : Fcn  Expr=sin(u(1))
  R21 : Fcn  Expr=-sin(u(1))
  R22 : Fcn  Expr=cos(u(1))
  Vector Concatenate6 : Concatenate
  Vector Concatenate7 : Concatenate
  Vector Concatenate8 : Concatenate  Mode=Multidimensional array  ConcatenateDimension=2
  Out1 : Outport  VectorParamsAs1DForOutWhenUnconnected=off
  wires:
  Vector Concatenate8/1 -> Out1/1
  R22/1 -> Vector Concatenate7/2
  R12/1 -> Vector Concatenate7/1
  R21/1 -> Vector Concatenate6/2
  R11/1 -> Vector Concatenate6/1
  Vector Concatenate7/1 -> Vector Concatenate8/2
  Vector Concatenate6/1 -> Vector Concatenate8/1
  Bus Selector/1 -> R22/1, R21/1, R12/1, R11/1  "<alpha>"
  In1/1 -> Bus Selector/1

== system CACC_4_Robots/Subsystem1/controllers/Switch Case Ext. LA/dz3,dz4 calculation/beta1 ==
  In1 : Inport
  Add : Sum
  Bus Selector2 : BusSelector  OutputSignals=alpha,v_ref,theta_ref  OutputAsBus=on
  Bus Selector3 : BusSelector  OutputSignals=theta_ref,thetadot_ref,s  OutputAsBus=on
  Fcn2 : Fcn  Expr=(1-cos(u(1)))*u(2)*cos(u(3))-sin(u(1))*u(2)*sin(u(3))
  Fcn3 : Fcn  Expr=sin(u(1))*u(2)*cos(u(3))+(1-cos(u(1)))*u(2)*sin(u(3))
  Fcn4 : Fcn  Expr=cos(u(1))*u(3)*u(2)
  Fcn5 : Fcn  Expr=sin(u(1))*u(3)*u(2)
  Mux3 : Mux  Inputs=2
  Mux4 : Mux  Inputs=2
  Out1 : Outport  VectorParamsAs1DForOutWhenUnconnected=off
  wires:
  Bus Selector2/1 -> Fcn3/1, Fcn2/1
  Fcn2/1 -> Mux3/1
  Fcn3/1 -> Mux3/2
  Bus Selector3/1 -> Fcn5/1, Fcn4/1
  Fcn4/1 -> Mux4/1
  Fcn5/1 -> Mux4/2
  Mux3/1 -> Add/1
  Mux4/1 -> Add/2
  In1/1 -> Bus Selector3/1, Bus Selector2/1
  Add/1 -> Out1/1

== system CACC_4_Robots/Subsystem1/controllers/Switch Case Ext. LA/dz3,dz4 calculation/beta2 ==
  In1 : Inport
  Bus Selector : BusSelector  OutputSignals=v,theta,alpha,curv  OutputAsBus=on
  Mux : Mux  Inputs=2
  beta2_1 : Fcn  Expr=-u(1)*sin(u(2)+u(3))*(h*u(4)*cos(u(3))^2)
  beta2_2 : Fcn  Expr=u(1)*cos(u(2)+u(3))*(h*u(4)*cos(u(3))^2)
  Out1 : Outport  VectorParamsAs1DForOutWhenUnconnected=off
  wires:
  In1/1 -> Bus Selector/1
  Bus Selector/1 -> beta2_2/1, beta2_1/1
  beta2_1/1 -> Mux/1
  beta2_2/1 -> Mux/2
  Mux/1 -> Out1/1

== system CACC_4_Robots/Subsystem1/controllers/Switch Case Ext. LA/dz3,dz4 calculation/eq Sig3 line 3 ==
  In1 : Inport
  1 : Fcn  Expr=u(1)*cos(u(2))
  2 : Fcn  Expr=u(1)*sin(u(2))
  Bus Selector1 : BusSelector  OutputSignals=v_ref,theta_ref  OutputAsBus=on
  Vector Concatenate3 : Concatenate
  mat : Subsystem
  Out1 : Outport  VectorParamsAs1DForOutWhenUnconnected=off
  v_i-1 : Outport  Port=2  VectorParamsAs1DForOutWhenUnconnected=off
  wires:
  In1/1 -> mat/1(In1), Bus Selector1/1
  Bus Selector1/1 -> 2/1, 1/1
  1/1 -> Vector Concatenate3/1
  2/1 -> Vector Concatenate3/2
  mat/1(Out1) -> Out1/1
  Vector Concatenate3/1 -> v_i-1/1

== system CACC_4_Robots/Subsystem1/controllers/Switch Case Ext. LA/s/Approximation of s around zero ==
  In1 : Inport
  Action Port : ActionPort  ActionPortLabel=if(u1 < 0.01 & u1 > -0.01)
  Taylor approximation 3rd order : Fcn  Expr=0.5*(r+h*u(2))^2*u(1)-0.125*(r+h*u(2))^4*u(1)^3
  Out1 : Outport  VectorParamsAs1DForOutWhenUnconnected=off
  wires:
  In1/1 -> Taylor approximation 3rd order/1
  Taylor approximation 3rd order/1 -> Out1/1

== system CACC_4_Robots/Subsystem1/controllers/Switch Case Ext. LA/s/function s ==
  In1 : Inport
  Action Port : ActionPort  ActionPortLabel=else
  function s : Fcn  Expr=(-1+sqrt(1+u(1)^2*(r+h*u(2))^2))/u(1)
  Out1 : Outport  VectorParamsAs1DForOutWhenUnconnected=off
  wires:
  In1/1 -> function s/1
  function s/1 -> Out1/1

== system CACC_4_Robots/Subsystem2/controllers/Switch Case Ext. LA/disturbance term simplified/GamInv  ==
  In1 : Inport
  11 : Fcn  Expr=(r+h*u(1))*cos(u(2))
  12 : Fcn  Expr=(r+h*u(1))*sin(u(2))
  21 : Fcn  Expr=-h*sin(u(2))-h*sin(u(13))*cos(u(8))
  22 : Fcn  Expr=h*cos(u(2))-h*sin(u(13))*sin(u(8))
  Divide{,1..3} (4 alike) : Product  Inputs=*/
  Vector Concatenate : Concatenate
  Vector Concatenate1 : Concatenate
  Vector Concatenate2 : Concatenate  Mode=Multidimensional array  ConcatenateDimension=2
  det(Gam) : Fcn  Expr=((r+h*u(1))*(h-h*sin(u(13))*sin(u(8)-u(2))))
  GamInv : Outport  VectorParamsAs1DForOutWhenUnconnected=off
  wires:
  Vector Concatenate2/1 -> GamInv/1
  Vector Concatenate1/1 -> Vector Concatenate2/2
  Vector Concatenate/1 -> Vector Concatenate2/1
  Divide3/1 -> Vector Concatenate1/2
  Divide1/1 -> Vector Concatenate1/1
  Divide2/1 -> Vector Concatenate/2
  Divide/1 -> Vector Concatenate/1
  In1/1 -> 11/1, 12/1, 21/1, 22/1, det(Gam)/1
  det(Gam)/1 -> Divide3/2, Divide/2, Divide1/2, Divide2/2
  22/1 -> Divide3/1
  21/1 -> Divide2/1
  12/1 -> Divide1/1
  11/1 -> Divide/1

== system CACC_4_Robots/Subsystem2/controllers/Switch Case Ext. LA/disturbance term simplified/H ==
  In1 : Inport
  Bus Selector1 : BusSelector  OutputSignals=v,theta  OutputAsBus=on
  H11 : Fcn  Expr=cos(u(2))
  H12 : Fcn  Expr=-u(1)*sin(u(2))
  H21 : Fcn  Expr=sin(u(2))
  H22 : Fcn  Expr=u(1)*cos(u(2))
  Vector Concatenate3 : Concatenate
  Vector Concatenate4 : Concatenate
  Vector Concatenate5 : Concatenate  Mode=Multidimensional array  ConcatenateDimension=2
  Out1 : Outport  VectorParamsAs1DForOutWhenUnconnected=off
  wires:
  Vector Concatenate5/1 -> Out1/1
  H22/1 -> Vector Concatenate4/2
  H12/1 -> Vector Concatenate4/1
  H21/1 -> Vector Concatenate3/2
  H11/1 -> Vector Concatenate3/1
  Vector Concatenate4/1 -> Vector Concatenate5/2
  Vector Concatenate3/1 -> Vector Concatenate5/1
  In1/1 -> Bus Selector1/1
  Bus Selector1/1 -> H12/1, H21/1, H22/1, H11/1

== system CACC_4_Robots/Subsystem2/controllers/Switch Case Ext. LA/disturbance term simplified/H1 ==
  In1 : Inport
  Bus Selector1 : BusSelector  OutputSignals=v,theta  OutputAsBus=on
  H11 : Fcn  Expr=cos(u(2))
  H12 : Fcn  Expr=-u(1)*sin(u(2))
  H21 : Fcn  Expr=sin(u(2))
  H22 : Fcn  Expr=u(1)*cos(u(2))
  Vector Concatenate3 : Concatenate
  Vector Concatenate4 : Concatenate
  Vector Concatenate5 : Concatenate  Mode=Multidimensional array  ConcatenateDimension=2
  Out1 : Outport  VectorParamsAs1DForOutWhenUnconnected=off
  wires:
  Bus Selector1/1 -> H11/1, H22/1, H21/1, H12/1
  In1/1 -> Bus Selector1/1
  Vector Concatenate3/1 -> Vector Concatenate5/1
  Vector Concatenate4/1 -> Vector Concatenate5/2
  H11/1 -> Vector Concatenate3/1
  H21/1 -> Vector Concatenate3/2
  H12/1 -> Vector Concatenate4/1
  H22/1 -> Vector Concatenate4/2
  Vector Concatenate5/1 -> Out1/1

== system CACC_4_Robots/Subsystem2/controllers/Switch Case Ext. LA/disturbance term simplified/R(alph) ==
  In1 : Inport
  Bus Selector : BusSelector  OutputSignals=alpha
  R11 : Fcn  Expr=cos(u(1))
  R12 : Fcn  Expr=-sin(u(1))
  R21 : Fcn  Expr=sin(u(1))
  R22 : Fcn  Expr=cos(u(1))
  Vector Concatenate6 : Concatenate
  Vector Concatenate7 : Concatenate
  Vector Concatenate8 : Concatenate  Mode=Multidimensional array  ConcatenateDimension=2
  Out1 : Outport  VectorParamsAs1DForOutWhenUnconnected=off
  wires:
  Vector Concatenate8/1 -> Out1/1
  R22/1 -> Vector Concatenate7/2
  R12/1 -> Vector Concatenate7/1
  R21/1 -> Vector Concatenate6/2
  R11/1 -> Vector Concatenate6/1
  Vector Concatenate7/1 -> Vector Concatenate8/2
  Vector Concatenate6/1 -> Vector Concatenate8/1
  Bus Selector/1 -> R22/1, R21/1, R12/1, R11/1  "<alpha>"
  In1/1 -> Bus Selector/1

== system CACC_4_Robots/Subsystem2/controllers/Switch Case Ext. LA/disturbance term simplified/beta1 ==
  In1 : Inport
  1 : Fcn  Expr=u(1)*cos(u(2))
  11 : Fcn  Expr=u(2)*(r+h*u(1))*sin(u(3))
  12 : Fcn  Expr=-sin(u(3))
  2 : Fcn  Expr=u(1)*sin(u(2))
  Bus Selector : BusSelector  OutputSignals=v,curv,alpha  OutputAsBus=on
  Bus Selector1 : BusSelector  OutputSignals=v_ref,theta_ref  OutputAsBus=on
  Product : Product  Multiplication=Matrix(*)
  Vector Concatenate : Concatenate
  Vector Concatenate1 : Concatenate
  Vector Concatenate2 : Concatenate  Mode=Multidimensional array  ConcatenateDimension=2
  Vector Concatenate3 : Concatenate
  Out1 : Outport  VectorParamsAs1DForOutWhenUnconnected=off
  wires:
  In1/1 -> Bus Selector1/1, Bus Selector/1
  Bus Selector/1 -> 11/1, 12/1
  11/1 -> Vector Concatenate1/2, Vector Concatenate/1
  12/1 -> Vector Concatenate1/1, Vector Concatenate/2
  Vector Concatenate/1 -> Vector Concatenate2/1
  Vector Concatenate1/1 -> Vector Concatenate2/2
  1/1 -> Vector Concatenate3/1
  2/1 -> Vector Concatenate3/2
  Bus Selector1/1 -> 2/1, 1/1
  Vector Concatenate2/1 -> Product/1
  Vector Concatenate3/1 -> Product/2
  Product/1 -> Out1/1

== system CACC_4_Robots/Subsystem2/controllers/Switch Case Ext. LA/dz3,dz4 calculation/GamInv  ==
  In1 : Inport
  11 : Fcn  Expr=(r+h*u(1))*cos(u(2))
  12 : Fcn  Expr=(r+h*u(1))*sin(u(2))
  21 : Fcn  Expr=-h*sin(u(2))-h*sin(u(13))*cos(u(8))
  22 : Fcn  Expr=h*cos(u(2))-h*sin(u(13))*sin(u(8))
  Divide{,1..3} (4 alike) : Product  Inputs=*/
  Vector Concatenate : Concatenate
  Vector Concatenate1 : Concatenate
  Vector Concatenate2 : Concatenate  Mode=Multidimensional array  ConcatenateDimension=2
  det(Gam) : Fcn  Expr=((r+h*u(1))*(h-h*sin(u(13))*sin(u(8)-u(2))))
  GamInv : Outport  VectorParamsAs1DForOutWhenUnconnected=off
  wires:
  11/1 -> Divide/1
  12/1 -> Divide1/1
  21/1 -> Divide2/1
  22/1 -> Divide3/1
  det(Gam)/1 -> Divide2/2, Divide1/2, Divide/2, Divide3/2
  In1/1 -> det(Gam)/1, 22/1, 21/1, 12/1, 11/1
  Divide/1 -> Vector Concatenate/1
  Divide2/1 -> Vector Concatenate/2
  Divide1/1 -> Vector Concatenate1/1
  Divide3/1 -> Vector Concatenate1/2
  Vector Concatenate/1 -> Vector Concatenate2/1
  Vector Concatenate1/1 -> Vector Concatenate2/2
  Vector Concatenate2/1 -> GamInv/1

== system CACC_4_Robots/Subsystem2/controllers/Switch Case Ext. LA/dz3,dz4 calculation/H_i ==
  In1 : Inport
  Bus Selector1 : BusSelector  OutputSignals=v,theta  OutputAsBus=on
  H11 : Fcn  Expr=cos(u(2))
  H12 : Fcn  Expr=-u(1)*sin(u(2))
  H21 : Fcn  Expr=sin(u(2))
  H22 : Fcn  Expr=u(1)*cos(u(2))
  Vector Concatenate3 : Concatenate
  Vector Concatenate4 : Concatenate
  Vector Concatenate5 : Concatenate  Mode=Multidimensional array  ConcatenateDimension=2
  Out1 : Outport  VectorParamsAs1DForOutWhenUnconnected=off
  wires:
  Bus Selector1/1 -> H11/1, H22/1, H21/1, H12/1
  In1/1 -> Bus Selector1/1
  Vector Concatenate3/1 -> Vector Concatenate5/1
  Vector Concatenate4/1 -> Vector Concatenate5/2
  H11/1 -> Vector Concatenate3/1
  H21/1 -> Vector Concatenate3/2
  H12/1 -> Vector Concatenate4/1
  H22/1 -> Vector Concatenate4/2
  Vector Concatenate5/1 -> Out1/1

== system CACC_4_Robots/Subsystem2/controllers/Switch Case Ext. LA/dz3,dz4 calculation/H_i-1 ==
  In1 : Inport
  Bus Selector1 : BusSelector  OutputSignals=v_ref,theta_ref  OutputAsBus=on
  H11 : Fcn  Expr=cos(u(2))
  H12 : Fcn  Expr=-u(1)*sin(u(2))
  H21 : Fcn  Expr=sin(u(2))
  H22 : Fcn  Expr=u(1)*cos(u(2))
  Vector Concatenate3 : Concatenate
  Vector Concatenate4 : Concatenate
  Vector Concatenate5 : Concatenate  Mode=Multidimensional array  ConcatenateDimension=2
  Out1 : Outport  VectorParamsAs1DForOutWhenUnconnected=off
  wires:
  Vector Concatenate5/1 -> Out1/1
  H22/1 -> Vector Concatenate4/2
  H12/1 -> Vector Concatenate4/1
  H21/1 -> Vector Concatenate3/2
  H11/1 -> Vector Concatenate3/1
  Vector Concatenate4/1 -> Vector Concatenate5/2
  Vector Concatenate3/1 -> Vector Concatenate5/1
  In1/1 -> Bus Selector1/1
  Bus Selector1/1 -> H12/1, H21/1, H22/1, H11/1

== system CACC_4_Robots/Subsystem2/controllers/Switch Case Ext. LA/dz3,dz4 calculation/R(alph) ==
  In1 : Inport
  Bus Selector : BusSelector  OutputSignals=alpha
  R11 : Fcn  Expr=cos(u(1))
  R12 : Fcn  Expr=-sin(u(1))
  R21 : Fcn  Expr=sin(u(1))
  R22 : Fcn  Expr=cos(u(1))
  Vector Concatenate6 : Concatenate
  Vector Concatenate7 : Concatenate
  Vector Concatenate8 : Concatenate  Mode=Multidimensional array  ConcatenateDimension=2
  Out1 : Outport  VectorParamsAs1DForOutWhenUnconnected=off
  wires:
  In1/1 -> Bus Selector/1
  Bus Selector/1 -> R11/1, R12/1, R21/1, R22/1  "<alpha>"
  Vector Concatenate6/1 -> Vector Concatenate8/1
  Vector Concatenate7/1 -> Vector Concatenate8/2
  R11/1 -> Vector Concatenate6/1
  R21/1 -> Vector Concatenate6/2
  R12/1 -> Vector Concatenate7/1
  R22/1 -> Vector Concatenate7/2
  Vector Concatenate8/1 -> Out1/1

== system CACC_4_Robots/Subsystem2/controllers/Switch Case Ext. LA/dz3,dz4 calculation/Rinv(alph) ==
  In1 : Inport
  Bus Selector : BusSelector  OutputSignals=alpha
  R11 : Fcn  Expr=cos(u(1))
  R12 : Fcn  Expr=sin(u(1))
  R21 : Fcn  Expr=-sin(u(1))
  R22 : Fcn  Expr=cos(u(1))
  Vector Concatenate6 : Concatenate
  Vector Concatenate7 : Concatenate
  Vector Concatenate8 : Concatenate  Mode=Multidimensional array  ConcatenateDimension=2
  Out1 : Outport  VectorParamsAs1DForOutWhenUnconnected=off
  wires:
  Vector Concatenate8/1 -> Out1/1
  R22/1 -> Vector Concatenate7/2
  R12/1 -> Vector Concatenate7/1
  R21/1 -> Vector Concatenate6/2
  R11/1 -> Vector Concatenate6/1
  Vector Concatenate7/1 -> Vector Concatenate8/2
  Vector Concatenate6/1 -> Vector Concatenate8/1
  Bus Selector/1 -> R22/1, R21/1, R12/1, R11/1  "<alpha>"
  In1/1 -> Bus Selector/1

== system CACC_4_Robots/Subsystem2/controllers/Switch Case Ext. LA/dz3,dz4 calculation/beta1 ==
  In1 : Inport
  Add : Sum
  Bus Selector2 : BusSelector  OutputSignals=alpha,v_ref,theta_ref  OutputAsBus=on
  Bus Selector3 : BusSelector  OutputSignals=theta_ref,thetadot_ref,s  OutputAsBus=on
  Fcn2 : Fcn  Expr=(1-cos(u(1)))*u(2)*cos(u(3))-sin(u(1))*u(2)*sin(u(3))
  Fcn3 : Fcn  Expr=sin(u(1))*u(2)*cos(u(3))+(1-cos(u(1)))*u(2)*sin(u(3))
  Fcn4 : Fcn  Expr=cos(u(1))*u(3)*u(2)
  Fcn5 : Fcn  Expr=sin(u(1))*u(3)*u(2)
  Mux3 : Mux  Inputs=2
  Mux4 : Mux  Inputs=2
  Out1 : Outport  VectorParamsAs1DForOutWhenUnconnected=off
  wires:
  Bus Selector2/1 -> Fcn3/1, Fcn2/1
  Fcn2/1 -> Mux3/1
  Fcn3/1 -> Mux3/2
  Bus Selector3/1 -> Fcn5/1, Fcn4/1
  Fcn4/1 -> Mux4/1
  Fcn5/1 -> Mux4/2
  Mux3/1 -> Add/1
  Mux4/1 -> Add/2
  In1/1 -> Bus Selector3/1, Bus Selector2/1
  Add/1 -> Out1/1

== system CACC_4_Robots/Subsystem2/controllers/Switch Case Ext. LA/dz3,dz4 calculation/beta2 ==
  In1 : Inport
  Bus Selector : BusSelector  OutputSignals=v,theta,alpha,curv  OutputAsBus=on
  Mux : Mux  Inputs=2
  beta2_1 : Fcn  Expr=-u(1)*sin(u(2)+u(3))*(h*u(4)*cos(u(3))^2)
  beta2_2 : Fcn  Expr=u(1)*cos(u(2)+u(3))*(h*u(4)*cos(u(3))^2)
  Out1 : Outport  VectorParamsAs1DForOutWhenUnconnected=off
  wires:
  In1/1 -> Bus Selector/1
  Bus Selector/1 -> beta2_2/1, beta2_1/1
  beta2_1/1 -> Mux/1
  beta2_2/1 -> Mux/2
  Mux/1 -> Out1/1

== system CACC_4_Robots/Subsystem2/controllers/Switch Case Ext. LA/dz3,dz4 calculation/eq Sig3 line 3 ==
  In1 : Inport
  1 : Fcn  Expr=u(1)*cos(u(2))
  2 : Fcn  Expr=u(1)*sin(u(2))
  Bus Selector1 : BusSelector  OutputSignals=v_ref,theta_ref  OutputAsBus=on
  Vector Concatenate3 : Concatenate
  mat : Subsystem
  Out1 : Outport  VectorParamsAs1DForOutWhenUnconnected=off
  v_i-1 : Outport  Port=2  VectorParamsAs1DForOutWhenUnconnected=off
  wires:
  In1/1 -> mat/1(In1), Bus Selector1/1
  Bus Selector1/1 -> 2/1, 1/1
  1/1 -> Vector Concatenate3/1
  2/1 -> Vector Concatenate3/2
  mat/1(Out1) -> Out1/1
  Vector Concatenate3/1 -> v_i-1/1
